simulink subsystem "discrete_lqr_controller"  (R2025a)
settings: Solver=VariableStepAuto  StartTime=0.0  StopTime=10.0  RelTol=1e-3
values from neighbouring files (symbols this model uses):
  Ki_d = Kd(:, 13:15)    [constants.m]
  Kp_d = Kd(:, 1:12)    [constants.m]
settings Model: Creator=johnpye  LastModifiedBy=johnpye

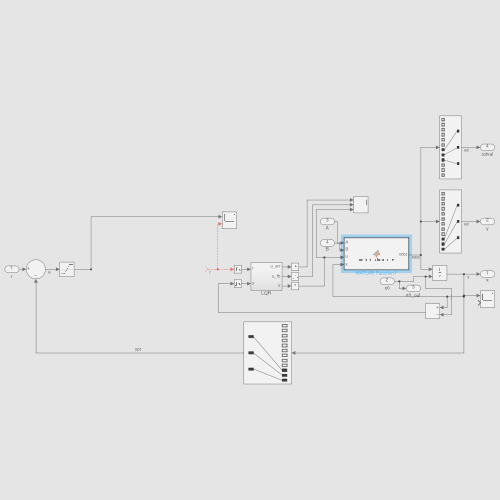
[thumbnail: Simulink's stored preview of the top-level diagram]
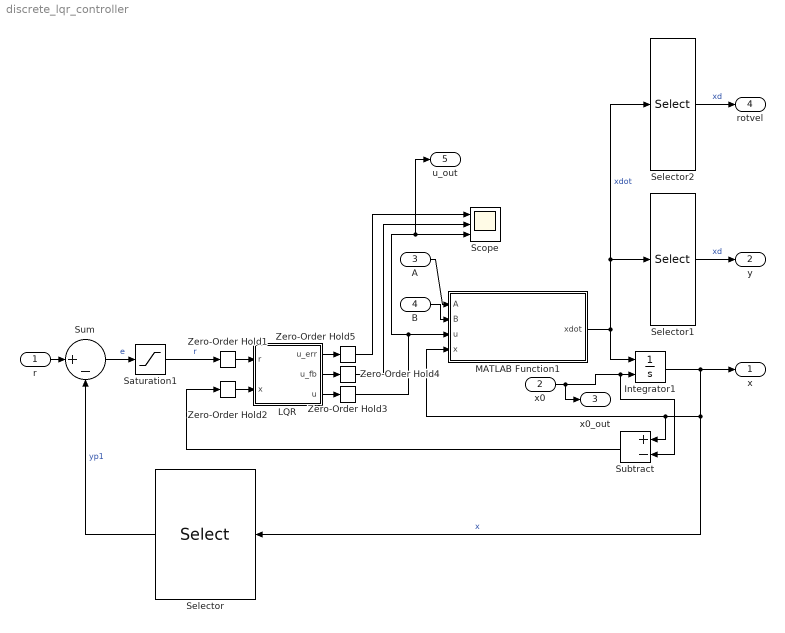
== system discrete_lqr_controller ==
  r : Inport
  x0 : Inport  Port=2
  A : Inport  Port=3
  B : Inport  Port=4
  Integrator1 : Integrator  InitialConditionSource=external  InitialCondition=[0; 0; 0; 0; 0; 0; 0; 0; 0; -1; 0; 0]
  LQR : Subsystem
  MATLAB Function1 : MATLAB Function  TreatAsAtomicUnit=on
  Saturation1 : Saturate  UpperLimit=[10; 10; 10]  LowerLimit=[-10; -10; -10]
  Scope : Scope  NumInputPorts=3
      settings: ActiveDisplayYMinimum=-1.0009054081910192E+10  ActiveDisplayYMaximum=1.3756629951484056E+9  DataLoggingVariableName=ScopeData28
  Selector : Selector  InputPortWidth=12  IndexOptions=Index vector (dialog)  Indices=[10 11 12]  OutputSizes=1
  Selector1 : Selector  InputPortWidth=12  IndexOptions=Index vector (dialog)  Indices=[10 11 12]  OutputSizes=1
  Selector2 : Selector  InputPortWidth=12  IndexOptions=Index vector (dialog)  Indices=[7 8 9]  OutputSizes=1
  Subtract : Sum  Inputs=+-
  Sum : Sum  Inputs=|+-
  Zero-Order Hold{1..5} (5 alike) : ZeroOrderHold  SampleTime=1/50
  x : Outport
  y : Outport  Port=2
  x0_out : Outport  Port=3
  rotvel : Outport  Port=4
  u_out : Outport  Port=5
  wires:
  A/1 -> MATLAB Function1/1(A)
  Integrator1/1 -> Selector/1, MATLAB Function1/4(x), Subtract/1, x/1  "x"
  Selector/1 -> Sum/2  "yp1"
  MATLAB Function1/1(xdot) -> Selector2/1, Selector1/1, Integrator1/1  "xdot"
  B/1 -> MATLAB Function1/2(B)
  Selector1/1 -> y/1  "xd"
  x0/1 -> x0_out/1, Subtract/2, Integrator1/2
  r/1 -> Sum/1
  Saturation1/1 -> Zero-Order Hold1/1  "r"
  Sum/1 -> Saturation1/1  "e"
  Selector2/1 -> rotvel/1  "xd"
  LQR/3(u) -> Zero-Order Hold3/1
  Subtract/1 -> Zero-Order Hold2/1
  LQR/1(u_err) -> Zero-Order Hold5/1
  LQR/2(u_fb) -> Zero-Order Hold4/1
  Zero-Order Hold1/1 -> LQR/1(r)
  Zero-Order Hold2/1 -> LQR/2(x)
  Zero-Order Hold3/1 -> MATLAB Function1/3(u), Scope/3, u_out/1
  Zero-Order Hold4/1 -> Scope/2
  Zero-Order Hold5/1 -> Scope/1

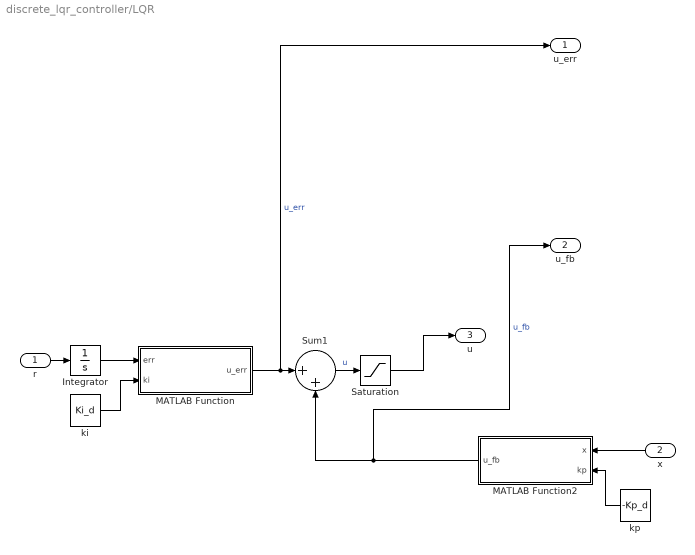
== system discrete_lqr_controller/LQR ==
  r : Inport
  x : Inport  Port=2
  Integrator : Integrator
  MATLAB Function : MATLAB Function  TreatAsAtomicUnit=on
  MATLAB Function2 : MATLAB Function  TreatAsAtomicUnit=on
  Saturation : Saturate  UpperLimit=[50; 0.3; 0.3; 0.3]  LowerLimit=-1*[50; 0.3; 0.3; 0.3]
  Sum1 : Sum  Inputs=|++
  ki : Constant  Value=Ki_d
  kp : Constant  Value=-Kp_d
  u_err : Outport
  u_fb : Outport  Port=2
  u : Outport  Port=3
  wires:
  x/1 -> MATLAB Function2/1(x)
  Saturation/1 -> u/1
  ki/1 -> MATLAB Function/2(ki)
  r/1 -> Integrator/1
  MATLAB Function/1(u_err) -> u_err/1, Sum1/1  "u_err"
  Integrator/1 -> MATLAB Function/1(err)
  kp/1 -> MATLAB Function2/2(kp)
  MATLAB Function2/1(u_fb) -> u_fb/1, Sum1/2  "u_fb"
  Sum1/1 -> Saturation/1  "u"

== matlab function discrete_lqr_controller/LQR/MATLAB Function ==
  data: err input; u_err output; ki input
function u_err = int_control(err, ki)

err = reshape(err, [3, 1]);
u_err = ki * err;

== matlab function discrete_lqr_controller/LQR/MATLAB Function2 ==
  data: x input; u_fb output; kp input
function u_fb = fb_control(x, kp)

x = reshape(x, [12, 1]);
u_fb = kp * x;

== matlab function discrete_lqr_controller/MATLAB Function1 ==
  data: A input; B input; u input; x input; xdot output
% function xdot = system_dynamics(A, B, u, x)
% 
% g = 9.81; % m/s^2
% l = 0.2; % m
% Jmp = 0;
% Jxx = 1.8e-3; % kgm^2
% Jyy = 1.8e-3; % kgm^2
% Jzz = 1.5e-3; % kgm^2
% kmt = 0.1; % m
% 
% K = B(4,2)*Jxx;
% m = (1/B(3,1)) * -K;
% 
% u = reshape(u, [4, 1]);
% u(1) = u(1) + 9.81*0.8;
% x = reshape(x, [12, 1]);
% % xdot = A*x + B*u;
% xdot=zeros(12,1);
% 
% vx = x(1);
% vy = x(2);
% vz = x(3);
% wx = x(4);
% wy = x(5);
% wz = x(6);
% theta = x(7);
% phi = x(8);
% psi = x(9);
% x = x(10);
% T = u(1);
% Mx = u(2);
% My = u(3);
% Mz = u(4);
% 
% % Step 3: Calculate derivatives
% xdot(1)         = -vz*wy + vy*wz - g*sin(theta);
% xdot(2)         = -vx*wz + vz*wx + g*cos(theta)*sin(phi);
% xdot(3)         = -vy*wx + vx*wy + g*cos(theta)*cos(phi) - T/m;
% xdot(4)         = (1/Jxx)*(-wy*wz*(Jzz - Jyy) + Mx);
% xdot(5)         = (1/Jyy)*(-wx*wz*(Jxx - Jzz) + My);
% xdot(6)         = Mz / Jzz;
% xdot(7)         = wy*cos(phi) - wz*sin(phi);
% xdot(8)         = wx + wy*sin(phi)*tan(theta) + wz*cos(phi)*tan(theta);
% xdot(9)         = wy*(sin(phi)/cos(theta)) + wz*(cos(phi)/cos(theta));
% xdot(10)        = vx*cos(psi)*cos(theta) + ...
%                     vy*(-sin(psi)*cos(phi) + cos(psi)*sin(theta)*sin(phi)) + ...
%                     vz*(sin(psi)*sin(phi) + cos(psi)*sin(theta)*cos(phi));
% xdot(11)        = vx*sin(psi)*cos(theta) + ...
%                     vy*(cos(psi)*cos(phi) + sin(psi)*sin(theta)*sin(phi)) + ...
%                     vz*(-cos(psi)*sin(phi) + sin(psi)*sin(theta)*cos(phi));
% xdot(12)        = vx*sin(theta) - vy*cos(theta)*sin(phi) - vz*cos(theta)*cos(phi);

function xdot = system_dynamics(A, B, u, x)

g = 9.81; % m/s^2
l = 0.2; % m
Jmp = 1e-5; % kgm^2
Jxx = 1.8e-3; % kgm^2
Jyy = 1.8e-3; % kgm^2
Jzz = 1.5e-3; % kgm^2
kmt = 0.1; % m
kwt = 0.1;

K = B(4,2)*Jxx;
m = (1/B(3,1)) * -K;

u = reshape(u, [4, 1]);
u(1) = u(1) + 9.81*0.8;
x = reshape(x, [12, 1]);
xdot=zeros(12,1);

vx = x(1);
vy = x(2);
vz = x(3);
wx = x(4);
wy = x(5);
wz = x(6);
theta = x(7);
phi = x(8);
psi = x(9);
% T = K*u(1);
% Mx = K*u(2);
% My = K*u(3);
% Mz = K*u(4);
T = u(1);
Mx = u(2);
My = u(3);
Mz = u(4);

% Step 3: Calculate derivatives
xdot(1)         = -vz*wy + vy*wz - g*sin(theta);
xdot(2)         = -vx*wz + vz*wx + g*cos(theta)*sin(phi);
xdot(3)         = -vy*wx + vx*wy + g*cos(theta)*cos(phi) - T/m;
xdot(4)         = (1/Jxx)*(-wy*wz*(Jzz - Jyy) + Mx - (kwt/kmt)*Jmp*Mz*wy);
xdot(5)         = (1/Jyy)*(-wx*wz*(Jxx - Jzz) + My - (kwt/kmt)*Jmp*Mz*wx);
xdot(6)         = Mz / Jzz;
xdot(7)         = wy*cos(phi) - wz*sin(phi);
xdot(8)         = wx + wy*sin(phi)*tan(theta) + wz*cos(phi)*tan(theta);
xdot(9)         = wy*(sin(phi)/cos(theta)) + wz*(cos(phi)/cos(theta));
xdot(10)        = vx*cos(psi)*cos(theta) + ...
                    vy*(-sin(psi)*cos(phi) + cos(psi)*sin(theta)*sin(phi)) + ...
                    vz*(sin(psi)*sin(phi) + cos(psi)*sin(theta)*cos(phi));
xdot(11)        = vx*sin(psi)*cos(theta) + ...
                    vy*(cos(psi)*cos(phi) + sin(psi)*sin(theta)*sin(phi)) + ...
                    vz*(-cos(psi)*sin(phi) + sin(psi)*sin(theta)*cos(phi));
xdot(12)        = vx*sin(theta) - vy*cos(theta)*sin(phi) - vz*cos(theta)*cos(phi);
